simulink model "COSTEP_Auto"  (R2024b)
settings: Solver=FixedStepAuto  StartTime=0.0  StopTime=25  FixedStep=1/3600  RelTol=1e-3
model workspace (MAT data in the model file):
  AD : Simulink.Parameter (value not decoded)
  AG : Simulink.Parameter (value not decoded)
  AH : Simulink.Parameter (value not decoded)
  AV : Simulink.Parameter (value not decoded)
  AVP : Simulink.Parameter (value not decoded)
  BCHL : Simulink.Parameter (value not decoded)
  BCHV : Simulink.Parameter (value not decoded)
  BD : Simulink.Parameter (value not decoded)
  BG : Simulink.Parameter (value not decoded)
  BH : Simulink.Parameter (value not decoded)
  BVP : Simulink.Parameter (value not decoded)
  CD : Simulink.Parameter (value not decoded)
  CG : Simulink.Parameter (value not decoded)
  CH : Simulink.Parameter (value not decoded)
  CVP : Simulink.Parameter (value not decoded)
  ISV : Simulink.Parameter (value not decoded)
  XMW : Simulink.Parameter (value not decoded)
  XNS : Simulink.Parameter (value not decoded)
  XNS2 : Simulink.Parameter (value not decoded)
  XNS3 : Simulink.Parameter (value not decoded)
  XNSE : Simulink.Parameter (value not decoded)
values from neighbouring files (symbols this model uses):
  DD = SimData{4,1}{1,2}    [Auto_run_COSTEP.m]    (also in Run_COSTEP.m)
  G = SimData{2,1}(j,2)    [Auto_run_COSTEP.m]    (also in G.mat = [4243534565 7854912354 3456432354 1731738903 4346024432 5784; Run_COSTEP.m)
  IDV = SimData{3,1}(1:20,j)    [Auto_run_COSTEP.m]    (also in IDV.mat = [0 0 0 0 0 0 0 0 0 0 0 0 ... (812 elements, 28x29)]; Run_COSTEP.m = SimData{3,1}(1:28,j))
symbols that are objects in the model workspace (value not decoded): AD, AG, AH, AV, AVP, BD, BG, BH, BVP, CD, CG, CH, CVP, XMW, XNS, XNS2, XNS3, XNSE
undefined symbols (not defined in the file or in its folder): magnitude, msgbox, SETPT, XMEAS, XMV
libraries: mylib x304, dspindex x31
(part 12 of 13)

== system COSTEP_Auto/Random number generator/Stream Measurements SMEAS Gas analysis/If Action Subsystem3/Subsystem/Stream 13/Subsystem/TESUB6 XMNSEH ==
  G : Inport
  Process Noise I=1-12 G New : mylib/Process Noise I=1-12 G New  SystemSampleTime=-1  VariantActivationTime=update diagram  AllowFlexibleInterface=on  Latency=0  AutoFrameSizeCalculation=off
  XNSEH : Constant  Value=0.05
  XMNSEH : Outport  VectorParamsAs1DForOutWhenUnconnected=off
  G_NEW : Outport  Port=2  VectorParamsAs1DForOutWhenUnconnected=off
  wires:
  XNSEH/1 -> Process Noise I=1-12 G New/1
  Process Noise I=1-12 G New/1 -> XMNSEH/1
  G/1 -> Process Noise I=1-12 G New/2
  Process Noise I=1-12 G New/2 -> G_NEW/1

== system COSTEP_Auto/Random number generator/Stream Measurements SMEAS Gas analysis/If Action Subsystem3/Subsystem/Stream 2/Subsystem/TESUB6 XMNSEA ==
  G : Inport
  Process Noise I=1-12 G New : mylib/Process Noise I=1-12 G New  SystemSampleTime=-1  VariantActivationTime=update diagram  AllowFlexibleInterface=on  Latency=0  AutoFrameSizeCalculation=off
  XNSEA : Constant  Value=0.25
  XMNSEA : Outport  VectorParamsAs1DForOutWhenUnconnected=off
  G_NEW : Outport  Port=2  VectorParamsAs1DForOutWhenUnconnected=off
  wires:
  XNSEA/1 -> Process Noise I=1-12 G New/1
  Process Noise I=1-12 G New/1 -> XMNSEA/1
  G/1 -> Process Noise I=1-12 G New/2
  Process Noise I=1-12 G New/2 -> G_NEW/1

== system COSTEP_Auto/Random number generator/Stream Measurements SMEAS Gas analysis/If Action Subsystem3/Subsystem/Stream 2/Subsystem/TESUB6 XMNSEB ==
  G : Inport
  Process Noise I=1-12 G New : mylib/Process Noise I=1-12 G New  SystemSampleTime=-1  VariantActivationTime=update diagram  AllowFlexibleInterface=on  Latency=0  AutoFrameSizeCalculation=off
  XNSEB : Constant  Value=0.1
  XMNSEB : Outport  VectorParamsAs1DForOutWhenUnconnected=off
  G_NEW : Outport  Port=2  VectorParamsAs1DForOutWhenUnconnected=off
  wires:
  XNSEB/1 -> Process Noise I=1-12 G New/1
  Process Noise I=1-12 G New/1 -> XMNSEB/1
  G/1 -> Process Noise I=1-12 G New/2
  Process Noise I=1-12 G New/2 -> G_NEW/1

== system COSTEP_Auto/Random number generator/Stream Measurements SMEAS Gas analysis/If Action Subsystem3/Subsystem/Stream 2/Subsystem/TESUB6 XMNSEC ==
  G : Inport
  Process Noise I=1-12 G New : mylib/Process Noise I=1-12 G New  SystemSampleTime=-1  VariantActivationTime=update diagram  AllowFlexibleInterface=on  Latency=0  AutoFrameSizeCalculation=off
  XNSEC : Constant  Value=0.25
  XMNSEC : Outport  VectorParamsAs1DForOutWhenUnconnected=off
  G_NEW : Outport  Port=2  VectorParamsAs1DForOutWhenUnconnected=off
  wires:
  XNSEC/1 -> Process Noise I=1-12 G New/1
  Process Noise I=1-12 G New/1 -> XMNSEC/1
  G/1 -> Process Noise I=1-12 G New/2
  Process Noise I=1-12 G New/2 -> G_NEW/1

== system COSTEP_Auto/Random number generator/Stream Measurements SMEAS Gas analysis/If Action Subsystem3/Subsystem/Stream 2/Subsystem/TESUB6 XMNSED ==
  G : Inport
  Process Noise I=1-12 G New : mylib/Process Noise I=1-12 G New  SystemSampleTime=-1  VariantActivationTime=update diagram  AllowFlexibleInterface=on  Latency=0  AutoFrameSizeCalculation=off
  XNSED : Constant  Value=0.1
  XMNSED : Outport  VectorParamsAs1DForOutWhenUnconnected=off
  G_NEW : Outport  Port=2  VectorParamsAs1DForOutWhenUnconnected=off
  wires:
  XNSED/1 -> Process Noise I=1-12 G New/1
  Process Noise I=1-12 G New/1 -> XMNSED/1
  G/1 -> Process Noise I=1-12 G New/2
  Process Noise I=1-12 G New/2 -> G_NEW/1

== system COSTEP_Auto/Random number generator/Stream Measurements SMEAS Gas analysis/If Action Subsystem3/Subsystem/Stream 2/Subsystem/TESUB6 XMNSEE ==
  G : Inport
  Process Noise I=1-12 G New : mylib/Process Noise I=1-12 G New  SystemSampleTime=-1  VariantActivationTime=update diagram  AllowFlexibleInterface=on  Latency=0  AutoFrameSizeCalculation=off
  XNSEE : Constant  Value=0.25
  XMNSEE : Outport  VectorParamsAs1DForOutWhenUnconnected=off
  G_NEW : Outport  Port=2  VectorParamsAs1DForOutWhenUnconnected=off
  wires:
  XNSEE/1 -> Process Noise I=1-12 G New/1
  Process Noise I=1-12 G New/1 -> XMNSEE/1
  G/1 -> Process Noise I=1-12 G New/2
  Process Noise I=1-12 G New/2 -> G_NEW/1

== system COSTEP_Auto/Random number generator/Stream Measurements SMEAS Gas analysis/If Action Subsystem3/Subsystem/Stream 2/Subsystem/TESUB6 XMNSEF ==
  G : Inport
  Process Noise I=1-12 G New : mylib/Process Noise I=1-12 G New  SystemSampleTime=-1  VariantActivationTime=update diagram  AllowFlexibleInterface=on  Latency=0  AutoFrameSizeCalculation=off
  XNSEF : Constant  Value=0.025
  XMNSEF : Outport  VectorParamsAs1DForOutWhenUnconnected=off
  G_NEW : Outport  Port=2  VectorParamsAs1DForOutWhenUnconnected=off
  wires:
  XNSEF/1 -> Process Noise I=1-12 G New/1
  Process Noise I=1-12 G New/1 -> XMNSEF/1
  G/1 -> Process Noise I=1-12 G New/2
  Process Noise I=1-12 G New/2 -> G_NEW/1

== system COSTEP_Auto/Random number generator/Stream Measurements SMEAS Gas analysis/If Action Subsystem3/Subsystem/Stream 2/Subsystem/TESUB6 XMNSEG ==
  G : Inport
  Process Noise I=1-12 G New : mylib/Process Noise I=1-12 G New  SystemSampleTime=-1  VariantActivationTime=update diagram  AllowFlexibleInterface=on  Latency=0  AutoFrameSizeCalculation=off
  XNSEG : Constant  Value=0.05
  XMNSEG : Outport  VectorParamsAs1DForOutWhenUnconnected=off
  G_NEW : Outport  Port=2  VectorParamsAs1DForOutWhenUnconnected=off
  wires:
  XNSEG/1 -> Process Noise I=1-12 G New/1
  Process Noise I=1-12 G New/1 -> XMNSEG/1
  G/1 -> Process Noise I=1-12 G New/2
  Process Noise I=1-12 G New/2 -> G_NEW/1

== system COSTEP_Auto/Random number generator/Stream Measurements SMEAS Gas analysis/If Action Subsystem3/Subsystem/Stream 2/Subsystem/TESUB6 XMNSEH ==
  G : Inport
  Process Noise I=1-12 G New : mylib/Process Noise I=1-12 G New  SystemSampleTime=-1  VariantActivationTime=update diagram  AllowFlexibleInterface=on  Latency=0  AutoFrameSizeCalculation=off
  XNSEH : Constant  Value=0.05
  XMNSEH : Outport  VectorParamsAs1DForOutWhenUnconnected=off
  G_NEW : Outport  Port=2  VectorParamsAs1DForOutWhenUnconnected=off
  wires:
  XNSEH/1 -> Process Noise I=1-12 G New/1
  Process Noise I=1-12 G New/1 -> XMNSEH/1
  G/1 -> Process Noise I=1-12 G New/2
  Process Noise I=1-12 G New/2 -> G_NEW/1

== system COSTEP_Auto/Random number generator/Stream Measurements SMEAS Gas analysis/If Action Subsystem3/Subsystem/Stream 3/Subsystem/TESUB6 XMNSEA ==
  G : Inport
  Process Noise I=1-12 G New : mylib/Process Noise I=1-12 G New  SystemSampleTime=-1  VariantActivationTime=update diagram  AllowFlexibleInterface=on  Latency=0  AutoFrameSizeCalculation=off
  XNSEA : Constant  Value=0.25
  XMNSEA : Outport  VectorParamsAs1DForOutWhenUnconnected=off
  G_NEW : Outport  Port=2  VectorParamsAs1DForOutWhenUnconnected=off
  wires:
  XNSEA/1 -> Process Noise I=1-12 G New/1
  Process Noise I=1-12 G New/1 -> XMNSEA/1
  G/1 -> Process Noise I=1-12 G New/2
  Process Noise I=1-12 G New/2 -> G_NEW/1

== system COSTEP_Auto/Random number generator/Stream Measurements SMEAS Gas analysis/If Action Subsystem3/Subsystem/Stream 3/Subsystem/TESUB6 XMNSEB ==
  G : Inport
  Process Noise I=1-12 G New : mylib/Process Noise I=1-12 G New  SystemSampleTime=-1  VariantActivationTime=update diagram  AllowFlexibleInterface=on  Latency=0  AutoFrameSizeCalculation=off
  XNSEB : Constant  Value=0.1
  XMNSEB : Outport  VectorParamsAs1DForOutWhenUnconnected=off
  G_NEW : Outport  Port=2  VectorParamsAs1DForOutWhenUnconnected=off
  wires:
  XNSEB/1 -> Process Noise I=1-12 G New/1
  Process Noise I=1-12 G New/1 -> XMNSEB/1
  G/1 -> Process Noise I=1-12 G New/2
  Process Noise I=1-12 G New/2 -> G_NEW/1

== system COSTEP_Auto/Random number generator/Stream Measurements SMEAS Gas analysis/If Action Subsystem3/Subsystem/Stream 3/Subsystem/TESUB6 XMNSEC ==
  G : Inport
  Process Noise I=1-12 G New : mylib/Process Noise I=1-12 G New  SystemSampleTime=-1  VariantActivationTime=update diagram  AllowFlexibleInterface=on  Latency=0  AutoFrameSizeCalculation=off
  XNSEC : Constant  Value=0.25
  XMNSEC : Outport  VectorParamsAs1DForOutWhenUnconnected=off
  G_NEW : Outport  Port=2  VectorParamsAs1DForOutWhenUnconnected=off
  wires:
  XNSEC/1 -> Process Noise I=1-12 G New/1
  Process Noise I=1-12 G New/1 -> XMNSEC/1
  G/1 -> Process Noise I=1-12 G New/2
  Process Noise I=1-12 G New/2 -> G_NEW/1

== system COSTEP_Auto/Random number generator/Stream Measurements SMEAS Gas analysis/If Action Subsystem3/Subsystem/Stream 3/Subsystem/TESUB6 XMNSED ==
  G : Inport
  Process Noise I=1-12 G New : mylib/Process Noise I=1-12 G New  SystemSampleTime=-1  VariantActivationTime=update diagram  AllowFlexibleInterface=on  Latency=0  AutoFrameSizeCalculation=off
  XNSED : Constant  Value=0.1
  XMNSED : Outport  VectorParamsAs1DForOutWhenUnconnected=off
  G_NEW : Outport  Port=2  VectorParamsAs1DForOutWhenUnconnected=off
  wires:
  XNSED/1 -> Process Noise I=1-12 G New/1
  Process Noise I=1-12 G New/1 -> XMNSED/1
  G/1 -> Process Noise I=1-12 G New/2
  Process Noise I=1-12 G New/2 -> G_NEW/1

== system COSTEP_Auto/Random number generator/Stream Measurements SMEAS Gas analysis/If Action Subsystem3/Subsystem/Stream 3/Subsystem/TESUB6 XMNSEE ==
  G : Inport
  Process Noise I=1-12 G New : mylib/Process Noise I=1-12 G New  SystemSampleTime=-1  VariantActivationTime=update diagram  AllowFlexibleInterface=on  Latency=0  AutoFrameSizeCalculation=off
  XNSEE : Constant  Value=0.25
  XMNSEE : Outport  VectorParamsAs1DForOutWhenUnconnected=off
  G_NEW : Outport  Port=2  VectorParamsAs1DForOutWhenUnconnected=off
  wires:
  XNSEE/1 -> Process Noise I=1-12 G New/1
  Process Noise I=1-12 G New/1 -> XMNSEE/1
  G/1 -> Process Noise I=1-12 G New/2
  Process Noise I=1-12 G New/2 -> G_NEW/1

== system COSTEP_Auto/Random number generator/Stream Measurements SMEAS Gas analysis/If Action Subsystem3/Subsystem/Stream 3/Subsystem/TESUB6 XMNSEF ==
  G : Inport
  Process Noise I=1-12 G New : mylib/Process Noise I=1-12 G New  SystemSampleTime=-1  VariantActivationTime=update diagram  AllowFlexibleInterface=on  Latency=0  AutoFrameSizeCalculation=off
  XNSEF : Constant  Value=0.025
  XMNSEF : Outport  VectorParamsAs1DForOutWhenUnconnected=off
  G_NEW : Outport  Port=2  VectorParamsAs1DForOutWhenUnconnected=off
  wires:
  XNSEF/1 -> Process Noise I=1-12 G New/1
  Process Noise I=1-12 G New/1 -> XMNSEF/1
  G/1 -> Process Noise I=1-12 G New/2
  Process Noise I=1-12 G New/2 -> G_NEW/1

== system COSTEP_Auto/Random number generator/Stream Measurements SMEAS Gas analysis/If Action Subsystem3/Subsystem/Stream 3/Subsystem/TESUB6 XMNSEG ==
  G : Inport
  Process Noise I=1-12 G New : mylib/Process Noise I=1-12 G New  SystemSampleTime=-1  VariantActivationTime=update diagram  AllowFlexibleInterface=on  Latency=0  AutoFrameSizeCalculation=off
  XNSEG : Constant  Value=0.05
  XMNSEG : Outport  VectorParamsAs1DForOutWhenUnconnected=off
  G_NEW : Outport  Port=2  VectorParamsAs1DForOutWhenUnconnected=off
  wires:
  XNSEG/1 -> Process Noise I=1-12 G New/1
  Process Noise I=1-12 G New/1 -> XMNSEG/1
  G/1 -> Process Noise I=1-12 G New/2
  Process Noise I=1-12 G New/2 -> G_NEW/1

== system COSTEP_Auto/Random number generator/Stream Measurements SMEAS Gas analysis/If Action Subsystem3/Subsystem/Stream 3/Subsystem/TESUB6 XMNSEH ==
  G : Inport
  Process Noise I=1-12 G New : mylib/Process Noise I=1-12 G New  SystemSampleTime=-1  VariantActivationTime=update diagram  AllowFlexibleInterface=on  Latency=0  AutoFrameSizeCalculation=off
  XNSEH : Constant  Value=0.05
  XMNSEH : Outport  VectorParamsAs1DForOutWhenUnconnected=off
  G_NEW : Outport  Port=2  VectorParamsAs1DForOutWhenUnconnected=off
  wires:
  XNSEH/1 -> Process Noise I=1-12 G New/1
  Process Noise I=1-12 G New/1 -> XMNSEH/1
  G/1 -> Process Noise I=1-12 G New/2
  Process Noise I=1-12 G New/2 -> G_NEW/1

== system COSTEP_Auto/Random number generator/Stream Measurements SMEAS Gas analysis/If Action Subsystem3/Subsystem/Stream 4/Subsystem/TESUB6 XMNSEA ==
  G : Inport
  Process Noise I=1-12 G New : mylib/Process Noise I=1-12 G New  SystemSampleTime=-1  VariantActivationTime=update diagram  AllowFlexibleInterface=on  Latency=0  AutoFrameSizeCalculation=off
  XNSEA : Constant  Value=0.25
  XMNSEA : Outport  VectorParamsAs1DForOutWhenUnconnected=off
  G_NEW : Outport  Port=2  VectorParamsAs1DForOutWhenUnconnected=off
  wires:
  XNSEA/1 -> Process Noise I=1-12 G New/1
  Process Noise I=1-12 G New/1 -> XMNSEA/1
  G/1 -> Process Noise I=1-12 G New/2
  Process Noise I=1-12 G New/2 -> G_NEW/1

== system COSTEP_Auto/Random number generator/Stream Measurements SMEAS Gas analysis/If Action Subsystem3/Subsystem/Stream 4/Subsystem/TESUB6 XMNSEB ==
  G : Inport
  Process Noise I=1-12 G New : mylib/Process Noise I=1-12 G New  SystemSampleTime=-1  VariantActivationTime=update diagram  AllowFlexibleInterface=on  Latency=0  AutoFrameSizeCalculation=off
  XNSEB : Constant  Value=0.1
  XMNSEB : Outport  VectorParamsAs1DForOutWhenUnconnected=off
  G_NEW : Outport  Port=2  VectorParamsAs1DForOutWhenUnconnected=off
  wires:
  XNSEB/1 -> Process Noise I=1-12 G New/1
  Process Noise I=1-12 G New/1 -> XMNSEB/1
  G/1 -> Process Noise I=1-12 G New/2
  Process Noise I=1-12 G New/2 -> G_NEW/1

== system COSTEP_Auto/Random number generator/Stream Measurements SMEAS Gas analysis/If Action Subsystem3/Subsystem/Stream 4/Subsystem/TESUB6 XMNSEC ==
  G : Inport
  Process Noise I=1-12 G New : mylib/Process Noise I=1-12 G New  SystemSampleTime=-1  VariantActivationTime=update diagram  AllowFlexibleInterface=on  Latency=0  AutoFrameSizeCalculation=off
  XNSEC : Constant  Value=0.25
  XMNSEC : Outport  VectorParamsAs1DForOutWhenUnconnected=off
  G_NEW : Outport  Port=2  VectorParamsAs1DForOutWhenUnconnected=off
  wires:
  XNSEC/1 -> Process Noise I=1-12 G New/1
  Process Noise I=1-12 G New/1 -> XMNSEC/1
  G/1 -> Process Noise I=1-12 G New/2
  Process Noise I=1-12 G New/2 -> G_NEW/1

== system COSTEP_Auto/Random number generator/Stream Measurements SMEAS Gas analysis/If Action Subsystem3/Subsystem/Stream 4/Subsystem/TESUB6 XMNSED ==
  G : Inport
  Process Noise I=1-12 G New : mylib/Process Noise I=1-12 G New  SystemSampleTime=-1  VariantActivationTime=update diagram  AllowFlexibleInterface=on  Latency=0  AutoFrameSizeCalculation=off
  XNSED : Constant  Value=0.1
  XMNSED : Outport  VectorParamsAs1DForOutWhenUnconnected=off
  G_NEW : Outport  Port=2  VectorParamsAs1DForOutWhenUnconnected=off
  wires:
  XNSED/1 -> Process Noise I=1-12 G New/1
  Process Noise I=1-12 G New/1 -> XMNSED/1
  G/1 -> Process Noise I=1-12 G New/2
  Process Noise I=1-12 G New/2 -> G_NEW/1

== system COSTEP_Auto/Random number generator/Stream Measurements SMEAS Gas analysis/If Action Subsystem3/Subsystem/Stream 4/Subsystem/TESUB6 XMNSEE ==
  G : Inport
  Process Noise I=1-12 G New : mylib/Process Noise I=1-12 G New  SystemSampleTime=-1  VariantActivationTime=update diagram  AllowFlexibleInterface=on  Latency=0  AutoFrameSizeCalculation=off
  XNSEE : Constant  Value=0.25
  XMNSEE : Outport  VectorParamsAs1DForOutWhenUnconnected=off
  G_NEW : Outport  Port=2  VectorParamsAs1DForOutWhenUnconnected=off
  wires:
  XNSEE/1 -> Process Noise I=1-12 G New/1
  Process Noise I=1-12 G New/1 -> XMNSEE/1
  G/1 -> Process Noise I=1-12 G New/2
  Process Noise I=1-12 G New/2 -> G_NEW/1

== system COSTEP_Auto/Random number generator/Stream Measurements SMEAS Gas analysis/If Action Subsystem3/Subsystem/Stream 4/Subsystem/TESUB6 XMNSEF ==
  G : Inport
  Process Noise I=1-12 G New : mylib/Process Noise I=1-12 G New  SystemSampleTime=-1  VariantActivationTime=update diagram  AllowFlexibleInterface=on  Latency=0  AutoFrameSizeCalculation=off
  XNSEF : Constant  Value=0.025
  XMNSEF : Outport  VectorParamsAs1DForOutWhenUnconnected=off
  G_NEW : Outport  Port=2  VectorParamsAs1DForOutWhenUnconnected=off
  wires:
  XNSEF/1 -> Process Noise I=1-12 G New/1
  Process Noise I=1-12 G New/1 -> XMNSEF/1
  G/1 -> Process Noise I=1-12 G New/2
  Process Noise I=1-12 G New/2 -> G_NEW/1

== system COSTEP_Auto/Random number generator/Stream Measurements SMEAS Gas analysis/If Action Subsystem3/Subsystem/Stream 4/Subsystem/TESUB6 XMNSEG ==
  G : Inport
  Process Noise I=1-12 G New : mylib/Process Noise I=1-12 G New  SystemSampleTime=-1  VariantActivationTime=update diagram  AllowFlexibleInterface=on  Latency=0  AutoFrameSizeCalculation=off
  XNSEG : Constant  Value=0.05
  XMNSEG : Outport  VectorParamsAs1DForOutWhenUnconnected=off
  G_NEW : Outport  Port=2  VectorParamsAs1DForOutWhenUnconnected=off
  wires:
  XNSEG/1 -> Process Noise I=1-12 G New/1
  Process Noise I=1-12 G New/1 -> XMNSEG/1
  G/1 -> Process Noise I=1-12 G New/2
  Process Noise I=1-12 G New/2 -> G_NEW/1

== system COSTEP_Auto/Random number generator/Stream Measurements SMEAS Gas analysis/If Action Subsystem3/Subsystem/Stream 4/Subsystem/TESUB6 XMNSEH ==
  G : Inport
  Process Noise I=1-12 G New : mylib/Process Noise I=1-12 G New  SystemSampleTime=-1  VariantActivationTime=update diagram  AllowFlexibleInterface=on  Latency=0  AutoFrameSizeCalculation=off
  XNSEH : Constant  Value=0.05
  XMNSEH : Outport  VectorParamsAs1DForOutWhenUnconnected=off
  G_NEW : Outport  Port=2  VectorParamsAs1DForOutWhenUnconnected=off
  wires:
  XNSEH/1 -> Process Noise I=1-12 G New/1
  Process Noise I=1-12 G New/1 -> XMNSEH/1
  G/1 -> Process Noise I=1-12 G New/2
  Process Noise I=1-12 G New/2 -> G_NEW/1

== system COSTEP_Auto/Random number generator/Stream Measurements SMEAS Gas analysis/If Action Subsystem3/Subsystem/Stream 5/Subsystem/TESUB6 XMNSEA ==
  G : Inport
  Process Noise I=1-12 G New : mylib/Process Noise I=1-12 G New  SystemSampleTime=-1  VariantActivationTime=update diagram  AllowFlexibleInterface=on  Latency=0  AutoFrameSizeCalculation=off
  XNSEA : Constant  Value=0.25
  XMNSEA : Outport  VectorParamsAs1DForOutWhenUnconnected=off
  G_NEW : Outport  Port=2  VectorParamsAs1DForOutWhenUnconnected=off
  wires:
  XNSEA/1 -> Process Noise I=1-12 G New/1
  Process Noise I=1-12 G New/1 -> XMNSEA/1
  G/1 -> Process Noise I=1-12 G New/2
  Process Noise I=1-12 G New/2 -> G_NEW/1

== system COSTEP_Auto/Random number generator/Stream Measurements SMEAS Gas analysis/If Action Subsystem3/Subsystem/Stream 5/Subsystem/TESUB6 XMNSEB ==
  G : Inport
  Process Noise I=1-12 G New : mylib/Process Noise I=1-12 G New  SystemSampleTime=-1  VariantActivationTime=update diagram  AllowFlexibleInterface=on  Latency=0  AutoFrameSizeCalculation=off
  XNSEB : Constant  Value=0.1
  XMNSEB : Outport  VectorParamsAs1DForOutWhenUnconnected=off
  G_NEW : Outport  Port=2  VectorParamsAs1DForOutWhenUnconnected=off
  wires:
  XNSEB/1 -> Process Noise I=1-12 G New/1
  Process Noise I=1-12 G New/1 -> XMNSEB/1
  G/1 -> Process Noise I=1-12 G New/2
  Process Noise I=1-12 G New/2 -> G_NEW/1

== system COSTEP_Auto/Random number generator/Stream Measurements SMEAS Gas analysis/If Action Subsystem3/Subsystem/Stream 5/Subsystem/TESUB6 XMNSEC ==
  G : Inport
  Process Noise I=1-12 G New : mylib/Process Noise I=1-12 G New  SystemSampleTime=-1  VariantActivationTime=update diagram  AllowFlexibleInterface=on  Latency=0  AutoFrameSizeCalculation=off
  XNSEC : Constant  Value=0.25
  XMNSEC : Outport  VectorParamsAs1DForOutWhenUnconnected=off
  G_NEW : Outport  Port=2  VectorParamsAs1DForOutWhenUnconnected=off
  wires:
  XNSEC/1 -> Process Noise I=1-12 G New/1
  Process Noise I=1-12 G New/1 -> XMNSEC/1
  G/1 -> Process Noise I=1-12 G New/2
  Process Noise I=1-12 G New/2 -> G_NEW/1

== system COSTEP_Auto/Random number generator/Stream Measurements SMEAS Gas analysis/If Action Subsystem3/Subsystem/Stream 5/Subsystem/TESUB6 XMNSED ==
  G : Inport
  Process Noise I=1-12 G New : mylib/Process Noise I=1-12 G New  SystemSampleTime=-1  VariantActivationTime=update diagram  AllowFlexibleInterface=on  Latency=0  AutoFrameSizeCalculation=off
  XNSED : Constant  Value=0.1
  XMNSED : Outport  VectorParamsAs1DForOutWhenUnconnected=off
  G_NEW : Outport  Port=2  VectorParamsAs1DForOutWhenUnconnected=off
  wires:
  XNSED/1 -> Process Noise I=1-12 G New/1
  Process Noise I=1-12 G New/1 -> XMNSED/1
  G/1 -> Process Noise I=1-12 G New/2
  Process Noise I=1-12 G New/2 -> G_NEW/1

== system COSTEP_Auto/Random number generator/Stream Measurements SMEAS Gas analysis/If Action Subsystem3/Subsystem/Stream 5/Subsystem/TESUB6 XMNSEE ==
  G : Inport
  Process Noise I=1-12 G New : mylib/Process Noise I=1-12 G New  SystemSampleTime=-1  VariantActivationTime=update diagram  AllowFlexibleInterface=on  Latency=0  AutoFrameSizeCalculation=off
  XNSEE : Constant  Value=0.25
  XMNSEE : Outport  VectorParamsAs1DForOutWhenUnconnected=off
  G_NEW : Outport  Port=2  VectorParamsAs1DForOutWhenUnconnected=off
  wires:
  XNSEE/1 -> Process Noise I=1-12 G New/1
  Process Noise I=1-12 G New/1 -> XMNSEE/1
  G/1 -> Process Noise I=1-12 G New/2
  Process Noise I=1-12 G New/2 -> G_NEW/1

== system COSTEP_Auto/Random number generator/Stream Measurements SMEAS Gas analysis/If Action Subsystem3/Subsystem/Stream 5/Subsystem/TESUB6 XMNSEF ==
  G : Inport
  Process Noise I=1-12 G New : mylib/Process Noise I=1-12 G New  SystemSampleTime=-1  VariantActivationTime=update diagram  AllowFlexibleInterface=on  Latency=0  AutoFrameSizeCalculation=off
  XNSEF : Constant  Value=0.025
  XMNSEF : Outport  VectorParamsAs1DForOutWhenUnconnected=off
  G_NEW : Outport  Port=2  VectorParamsAs1DForOutWhenUnconnected=off
  wires:
  XNSEF/1 -> Process Noise I=1-12 G New/1
  Process Noise I=1-12 G New/1 -> XMNSEF/1
  G/1 -> Process Noise I=1-12 G New/2
  Process Noise I=1-12 G New/2 -> G_NEW/1

== system COSTEP_Auto/Random number generator/Stream Measurements SMEAS Gas analysis/If Action Subsystem3/Subsystem/Stream 5/Subsystem/TESUB6 XMNSEG ==
  G : Inport
  Process Noise I=1-12 G New : mylib/Process Noise I=1-12 G New  SystemSampleTime=-1  VariantActivationTime=update diagram  AllowFlexibleInterface=on  Latency=0  AutoFrameSizeCalculation=off
  XNSEG : Constant  Value=0.05
  XMNSEG : Outport  VectorParamsAs1DForOutWhenUnconnected=off
  G_NEW : Outport  Port=2  VectorParamsAs1DForOutWhenUnconnected=off
  wires:
  XNSEG/1 -> Process Noise I=1-12 G New/1
  Process Noise I=1-12 G New/1 -> XMNSEG/1
  G/1 -> Process Noise I=1-12 G New/2
  Process Noise I=1-12 G New/2 -> G_NEW/1

== system COSTEP_Auto/Random number generator/Stream Measurements SMEAS Gas analysis/If Action Subsystem3/Subsystem/Stream 5/Subsystem/TESUB6 XMNSEH ==
  G : Inport
  Process Noise I=1-12 G New : mylib/Process Noise I=1-12 G New  SystemSampleTime=-1  VariantActivationTime=update diagram  AllowFlexibleInterface=on  Latency=0  AutoFrameSizeCalculation=off
  XNSEH : Constant  Value=0.05
  XMNSEH : Outport  VectorParamsAs1DForOutWhenUnconnected=off
  G_NEW : Outport  Port=2  VectorParamsAs1DForOutWhenUnconnected=off
  wires:
  XNSEH/1 -> Process Noise I=1-12 G New/1
  Process Noise I=1-12 G New/1 -> XMNSEH/1
  G/1 -> Process Noise I=1-12 G New/2
  Process Noise I=1-12 G New/2 -> G_NEW/1

== system COSTEP_Auto/Random number generator/Stream Measurements SMEAS Gas analysis/If Action Subsystem3/Subsystem/Stream 6/Subsystem/TESUB6 XMNSEA ==
  G : Inport
  Process Noise I=1-12 G New : mylib/Process Noise I=1-12 G New  SystemSampleTime=-1  VariantActivationTime=update diagram  AllowFlexibleInterface=on  Latency=0  AutoFrameSizeCalculation=off
  XNSEA : Constant  Value=0.25
  XMNSEA : Outport  VectorParamsAs1DForOutWhenUnconnected=off
  G_NEW : Outport  Port=2  VectorParamsAs1DForOutWhenUnconnected=off
  wires:
  XNSEA/1 -> Process Noise I=1-12 G New/1
  Process Noise I=1-12 G New/1 -> XMNSEA/1
  G/1 -> Process Noise I=1-12 G New/2
  Process Noise I=1-12 G New/2 -> G_NEW/1

== system COSTEP_Auto/Random number generator/Stream Measurements SMEAS Gas analysis/If Action Subsystem3/Subsystem/Stream 6/Subsystem/TESUB6 XMNSEB ==
  G : Inport
  Process Noise I=1-12 G New : mylib/Process Noise I=1-12 G New  SystemSampleTime=-1  VariantActivationTime=update diagram  AllowFlexibleInterface=on  Latency=0  AutoFrameSizeCalculation=off
  XNSEB : Constant  Value=0.1
  XMNSEB : Outport  VectorParamsAs1DForOutWhenUnconnected=off
  G_NEW : Outport  Port=2  VectorParamsAs1DForOutWhenUnconnected=off
  wires:
  XNSEB/1 -> Process Noise I=1-12 G New/1
  Process Noise I=1-12 G New/1 -> XMNSEB/1
  G/1 -> Process Noise I=1-12 G New/2
  Process Noise I=1-12 G New/2 -> G_NEW/1

== system COSTEP_Auto/Random number generator/Stream Measurements SMEAS Gas analysis/If Action Subsystem3/Subsystem/Stream 6/Subsystem/TESUB6 XMNSEC ==
  G : Inport
  Process Noise I=1-12 G New : mylib/Process Noise I=1-12 G New  SystemSampleTime=-1  VariantActivationTime=update diagram  AllowFlexibleInterface=on  Latency=0  AutoFrameSizeCalculation=off
  XNSEC : Constant  Value=0.25
  XMNSEC : Outport  VectorParamsAs1DForOutWhenUnconnected=off
  G_NEW : Outport  Port=2  VectorParamsAs1DForOutWhenUnconnected=off
  wires:
  XNSEC/1 -> Process Noise I=1-12 G New/1
  Process Noise I=1-12 G New/1 -> XMNSEC/1
  G/1 -> Process Noise I=1-12 G New/2
  Process Noise I=1-12 G New/2 -> G_NEW/1

== system COSTEP_Auto/Random number generator/Stream Measurements SMEAS Gas analysis/If Action Subsystem3/Subsystem/Stream 6/Subsystem/TESUB6 XMNSED ==
  G : Inport
  Process Noise I=1-12 G New : mylib/Process Noise I=1-12 G New  SystemSampleTime=-1  VariantActivationTime=update diagram  AllowFlexibleInterface=on  Latency=0  AutoFrameSizeCalculation=off
  XNSED : Constant  Value=0.1
  XMNSED : Outport  VectorParamsAs1DForOutWhenUnconnected=off
  G_NEW : Outport  Port=2  VectorParamsAs1DForOutWhenUnconnected=off
  wires:
  XNSED/1 -> Process Noise I=1-12 G New/1
  Process Noise I=1-12 G New/1 -> XMNSED/1
  G/1 -> Process Noise I=1-12 G New/2
  Process Noise I=1-12 G New/2 -> G_NEW/1

== system COSTEP_Auto/Random number generator/Stream Measurements SMEAS Gas analysis/If Action Subsystem3/Subsystem/Stream 6/Subsystem/TESUB6 XMNSEE ==
  G : Inport
  Process Noise I=1-12 G New : mylib/Process Noise I=1-12 G New  SystemSampleTime=-1  VariantActivationTime=update diagram  AllowFlexibleInterface=on  Latency=0  AutoFrameSizeCalculation=off
  XNSEE : Constant  Value=0.25
  XMNSEE : Outport  VectorParamsAs1DForOutWhenUnconnected=off
  G_NEW : Outport  Port=2  VectorParamsAs1DForOutWhenUnconnected=off
  wires:
  XNSEE/1 -> Process Noise I=1-12 G New/1
  Process Noise I=1-12 G New/1 -> XMNSEE/1
  G/1 -> Process Noise I=1-12 G New/2
  Process Noise I=1-12 G New/2 -> G_NEW/1

== system COSTEP_Auto/Random number generator/Stream Measurements SMEAS Gas analysis/If Action Subsystem3/Subsystem/Stream 6/Subsystem/TESUB6 XMNSEF ==
  G : Inport
  Process Noise I=1-12 G New : mylib/Process Noise I=1-12 G New  SystemSampleTime=-1  VariantActivationTime=update diagram  AllowFlexibleInterface=on  Latency=0  AutoFrameSizeCalculation=off
  XNSEF : Constant  Value=0.025
  XMNSEF : Outport  VectorParamsAs1DForOutWhenUnconnected=off
  G_NEW : Outport  Port=2  VectorParamsAs1DForOutWhenUnconnected=off
  wires:
  XNSEF/1 -> Process Noise I=1-12 G New/1
  Process Noise I=1-12 G New/1 -> XMNSEF/1
  G/1 -> Process Noise I=1-12 G New/2
  Process Noise I=1-12 G New/2 -> G_NEW/1

== system COSTEP_Auto/Random number generator/Stream Measurements SMEAS Gas analysis/If Action Subsystem3/Subsystem/Stream 6/Subsystem/TESUB6 XMNSEG ==
  G : Inport
  Process Noise I=1-12 G New : mylib/Process Noise I=1-12 G New  SystemSampleTime=-1  VariantActivationTime=update diagram  AllowFlexibleInterface=on  Latency=0  AutoFrameSizeCalculation=off
  XNSEG : Constant  Value=0.05
  XMNSEG : Outport  VectorParamsAs1DForOutWhenUnconnected=off
  G_NEW : Outport  Port=2  VectorParamsAs1DForOutWhenUnconnected=off
  wires:
  XNSEG/1 -> Process Noise I=1-12 G New/1
  Process Noise I=1-12 G New/1 -> XMNSEG/1
  G/1 -> Process Noise I=1-12 G New/2
  Process Noise I=1-12 G New/2 -> G_NEW/1

== system COSTEP_Auto/Random number generator/Stream Measurements SMEAS Gas analysis/If Action Subsystem3/Subsystem/Stream 6/Subsystem/TESUB6 XMNSEH ==
  G : Inport
  Process Noise I=1-12 G New : mylib/Process Noise I=1-12 G New  SystemSampleTime=-1  VariantActivationTime=update diagram  AllowFlexibleInterface=on  Latency=0  AutoFrameSizeCalculation=off
  XNSEH : Constant  Value=0.05
  XMNSEH : Outport  VectorParamsAs1DForOutWhenUnconnected=off
  G_NEW : Outport  Port=2  VectorParamsAs1DForOutWhenUnconnected=off
  wires:
  XNSEH/1 -> Process Noise I=1-12 G New/1
  Process Noise I=1-12 G New/1 -> XMNSEH/1
  G/1 -> Process Noise I=1-12 G New/2
  Process Noise I=1-12 G New/2 -> G_NEW/1

== system COSTEP_Auto/Random number generator/Stream Measurements SMEAS Gas analysis/If Action Subsystem3/Subsystem/Stream 8/Subsystem/TESUB6 XMNSEA ==
  G : Inport
  Process Noise I=1-12 G New : mylib/Process Noise I=1-12 G New  SystemSampleTime=-1  VariantActivationTime=update diagram  AllowFlexibleInterface=on  Latency=0  AutoFrameSizeCalculation=off
  XNSEA : Constant  Value=0.25
  XMNSEA : Outport  VectorParamsAs1DForOutWhenUnconnected=off
  G_NEW : Outport  Port=2  VectorParamsAs1DForOutWhenUnconnected=off
  wires:
  XNSEA/1 -> Process Noise I=1-12 G New/1
  Process Noise I=1-12 G New/1 -> XMNSEA/1
  G/1 -> Process Noise I=1-12 G New/2
  Process Noise I=1-12 G New/2 -> G_NEW/1

== system COSTEP_Auto/Random number generator/Stream Measurements SMEAS Gas analysis/If Action Subsystem3/Subsystem/Stream 8/Subsystem/TESUB6 XMNSEB ==
  G : Inport
  Process Noise I=1-12 G New : mylib/Process Noise I=1-12 G New  SystemSampleTime=-1  VariantActivationTime=update diagram  AllowFlexibleInterface=on  Latency=0  AutoFrameSizeCalculation=off
  XNSEB : Constant  Value=0.1
  XMNSEB : Outport  VectorParamsAs1DForOutWhenUnconnected=off
  G_NEW : Outport  Port=2  VectorParamsAs1DForOutWhenUnconnected=off
  wires:
  XNSEB/1 -> Process Noise I=1-12 G New/1
  Process Noise I=1-12 G New/1 -> XMNSEB/1
  G/1 -> Process Noise I=1-12 G New/2
  Process Noise I=1-12 G New/2 -> G_NEW/1

== system COSTEP_Auto/Random number generator/Stream Measurements SMEAS Gas analysis/If Action Subsystem3/Subsystem/Stream 8/Subsystem/TESUB6 XMNSEC ==
  G : Inport
  Process Noise I=1-12 G New : mylib/Process Noise I=1-12 G New  SystemSampleTime=-1  VariantActivationTime=update diagram  AllowFlexibleInterface=on  Latency=0  AutoFrameSizeCalculation=off
  XNSEC : Constant  Value=0.25
  XMNSEC : Outport  VectorParamsAs1DForOutWhenUnconnected=off
  G_NEW : Outport  Port=2  VectorParamsAs1DForOutWhenUnconnected=off
  wires:
  XNSEC/1 -> Process Noise I=1-12 G New/1
  Process Noise I=1-12 G New/1 -> XMNSEC/1
  G/1 -> Process Noise I=1-12 G New/2
  Process Noise I=1-12 G New/2 -> G_NEW/1

== system COSTEP_Auto/Random number generator/Stream Measurements SMEAS Gas analysis/If Action Subsystem3/Subsystem/Stream 8/Subsystem/TESUB6 XMNSED ==
  G : Inport
  Process Noise I=1-12 G New : mylib/Process Noise I=1-12 G New  SystemSampleTime=-1  VariantActivationTime=update diagram  AllowFlexibleInterface=on  Latency=0  AutoFrameSizeCalculation=off
  XNSED : Constant  Value=0.1
  XMNSED : Outport  VectorParamsAs1DForOutWhenUnconnected=off
  G_NEW : Outport  Port=2  VectorParamsAs1DForOutWhenUnconnected=off
  wires:
  XNSED/1 -> Process Noise I=1-12 G New/1
  Process Noise I=1-12 G New/1 -> XMNSED/1
  G/1 -> Process Noise I=1-12 G New/2
  Process Noise I=1-12 G New/2 -> G_NEW/1

== system COSTEP_Auto/Random number generator/Stream Measurements SMEAS Gas analysis/If Action Subsystem3/Subsystem/Stream 8/Subsystem/TESUB6 XMNSEE ==
  G : Inport
  Process Noise I=1-12 G New : mylib/Process Noise I=1-12 G New  SystemSampleTime=-1  VariantActivationTime=update diagram  AllowFlexibleInterface=on  Latency=0  AutoFrameSizeCalculation=off
  XNSEE : Constant  Value=0.25
  XMNSEE : Outport  VectorParamsAs1DForOutWhenUnconnected=off
  G_NEW : Outport  Port=2  VectorParamsAs1DForOutWhenUnconnected=off
  wires:
  XNSEE/1 -> Process Noise I=1-12 G New/1
  Process Noise I=1-12 G New/1 -> XMNSEE/1
  G/1 -> Process Noise I=1-12 G New/2
  Process Noise I=1-12 G New/2 -> G_NEW/1

== system COSTEP_Auto/Random number generator/Stream Measurements SMEAS Gas analysis/If Action Subsystem3/Subsystem/Stream 8/Subsystem/TESUB6 XMNSEF ==
  G : Inport
  Process Noise I=1-12 G New : mylib/Process Noise I=1-12 G New  SystemSampleTime=-1  VariantActivationTime=update diagram  AllowFlexibleInterface=on  Latency=0  AutoFrameSizeCalculation=off
  XNSEF : Constant  Value=0.025
  XMNSEF : Outport  VectorParamsAs1DForOutWhenUnconnected=off
  G_NEW : Outport  Port=2  VectorParamsAs1DForOutWhenUnconnected=off
  wires:
  XNSEF/1 -> Process Noise I=1-12 G New/1
  Process Noise I=1-12 G New/1 -> XMNSEF/1
  G/1 -> Process Noise I=1-12 G New/2
  Process Noise I=1-12 G New/2 -> G_NEW/1

== system COSTEP_Auto/Random number generator/Stream Measurements SMEAS Gas analysis/If Action Subsystem3/Subsystem/Stream 8/Subsystem/TESUB6 XMNSEG ==
  G : Inport
  Process Noise I=1-12 G New : mylib/Process Noise I=1-12 G New  SystemSampleTime=-1  VariantActivationTime=update diagram  AllowFlexibleInterface=on  Latency=0  AutoFrameSizeCalculation=off
  XNSEG : Constant  Value=0.05
  XMNSEG : Outport  VectorParamsAs1DForOutWhenUnconnected=off
  G_NEW : Outport  Port=2  VectorParamsAs1DForOutWhenUnconnected=off
  wires:
  XNSEG/1 -> Process Noise I=1-12 G New/1
  Process Noise I=1-12 G New/1 -> XMNSEG/1
  G/1 -> Process Noise I=1-12 G New/2
  Process Noise I=1-12 G New/2 -> G_NEW/1

== system COSTEP_Auto/Random number generator/Stream Measurements SMEAS Gas analysis/If Action Subsystem3/Subsystem/Stream 8/Subsystem/TESUB6 XMNSEH ==
  G : Inport
  Process Noise I=1-12 G New : mylib/Process Noise I=1-12 G New  SystemSampleTime=-1  VariantActivationTime=update diagram  AllowFlexibleInterface=on  Latency=0  AutoFrameSizeCalculation=off
  XNSEH : Constant  Value=0.05
  XMNSEH : Outport  VectorParamsAs1DForOutWhenUnconnected=off
  G_NEW : Outport  Port=2  VectorParamsAs1DForOutWhenUnconnected=off
  wires:
  XNSEH/1 -> Process Noise I=1-12 G New/1
  Process Noise I=1-12 G New/1 -> XMNSEH/1
  G/1 -> Process Noise I=1-12 G New/2
  Process Noise I=1-12 G New/2 -> G_NEW/1

== system COSTEP_Auto/Random number generator/Stream Measurements SMEAS Gas analysis/If Action Subsystem3/Subsystem/Stream 9/Subsystem/TESUB6 XMNSEA ==
  G : Inport
  Process Noise I=1-12 G New : mylib/Process Noise I=1-12 G New  SystemSampleTime=-1  VariantActivationTime=update diagram  AllowFlexibleInterface=on  Latency=0  AutoFrameSizeCalculation=off
  XNSEA : Constant  Value=0.25
  XMNSEA : Outport  VectorParamsAs1DForOutWhenUnconnected=off
  G_NEW : Outport  Port=2  VectorParamsAs1DForOutWhenUnconnected=off
  wires:
  XNSEA/1 -> Process Noise I=1-12 G New/1
  Process Noise I=1-12 G New/1 -> XMNSEA/1
  G/1 -> Process Noise I=1-12 G New/2
  Process Noise I=1-12 G New/2 -> G_NEW/1

== system COSTEP_Auto/Random number generator/Stream Measurements SMEAS Gas analysis/If Action Subsystem3/Subsystem/Stream 9/Subsystem/TESUB6 XMNSEB ==
  G : Inport
  Process Noise I=1-12 G New : mylib/Process Noise I=1-12 G New  SystemSampleTime=-1  VariantActivationTime=update diagram  AllowFlexibleInterface=on  Latency=0  AutoFrameSizeCalculation=off
  XNSEB : Constant  Value=0.1
  XMNSEB : Outport  VectorParamsAs1DForOutWhenUnconnected=off
  G_NEW : Outport  Port=2  VectorParamsAs1DForOutWhenUnconnected=off
  wires:
  XNSEB/1 -> Process Noise I=1-12 G New/1
  Process Noise I=1-12 G New/1 -> XMNSEB/1
  G/1 -> Process Noise I=1-12 G New/2
  Process Noise I=1-12 G New/2 -> G_NEW/1

== system COSTEP_Auto/Random number generator/Stream Measurements SMEAS Gas analysis/If Action Subsystem3/Subsystem/Stream 9/Subsystem/TESUB6 XMNSEC ==
  G : Inport
  Process Noise I=1-12 G New : mylib/Process Noise I=1-12 G New  SystemSampleTime=-1  VariantActivationTime=update diagram  AllowFlexibleInterface=on  Latency=0  AutoFrameSizeCalculation=off
  XNSEC : Constant  Value=0.25
  XMNSEC : Outport  VectorParamsAs1DForOutWhenUnconnected=off
  G_NEW : Outport  Port=2  VectorParamsAs1DForOutWhenUnconnected=off
  wires:
  XNSEC/1 -> Process Noise I=1-12 G New/1
  Process Noise I=1-12 G New/1 -> XMNSEC/1
  G/1 -> Process Noise I=1-12 G New/2
  Process Noise I=1-12 G New/2 -> G_NEW/1

== system COSTEP_Auto/Random number generator/Stream Measurements SMEAS Gas analysis/If Action Subsystem3/Subsystem/Stream 9/Subsystem/TESUB6 XMNSED ==
  G : Inport
  Process Noise I=1-12 G New : mylib/Process Noise I=1-12 G New  SystemSampleTime=-1  VariantActivationTime=update diagram  AllowFlexibleInterface=on  Latency=0  AutoFrameSizeCalculation=off
  XNSED : Constant  Value=0.1
  XMNSED : Outport  VectorParamsAs1DForOutWhenUnconnected=off
  G_NEW : Outport  Port=2  VectorParamsAs1DForOutWhenUnconnected=off
  wires:
  XNSED/1 -> Process Noise I=1-12 G New/1
  Process Noise I=1-12 G New/1 -> XMNSED/1
  G/1 -> Process Noise I=1-12 G New/2
  Process Noise I=1-12 G New/2 -> G_NEW/1

== system COSTEP_Auto/Random number generator/Stream Measurements SMEAS Gas analysis/If Action Subsystem3/Subsystem/Stream 9/Subsystem/TESUB6 XMNSEE ==
  G : Inport
  Process Noise I=1-12 G New : mylib/Process Noise I=1-12 G New  SystemSampleTime=-1  VariantActivationTime=update diagram  AllowFlexibleInterface=on  Latency=0  AutoFrameSizeCalculation=off
  XNSEE : Constant  Value=0.25
  XMNSEE : Outport  VectorParamsAs1DForOutWhenUnconnected=off
  G_NEW : Outport  Port=2  VectorParamsAs1DForOutWhenUnconnected=off
  wires:
  XNSEE/1 -> Process Noise I=1-12 G New/1
  Process Noise I=1-12 G New/1 -> XMNSEE/1
  G/1 -> Process Noise I=1-12 G New/2
  Process Noise I=1-12 G New/2 -> G_NEW/1

== system COSTEP_Auto/Random number generator/Stream Measurements SMEAS Gas analysis/If Action Subsystem3/Subsystem/Stream 9/Subsystem/TESUB6 XMNSEF ==
  G : Inport
  Process Noise I=1-12 G New : mylib/Process Noise I=1-12 G New  SystemSampleTime=-1  VariantActivationTime=update diagram  AllowFlexibleInterface=on  Latency=0  AutoFrameSizeCalculation=off
  XNSEF : Constant  Value=0.025
  XMNSEF : Outport  VectorParamsAs1DForOutWhenUnconnected=off
  G_NEW : Outport  Port=2  VectorParamsAs1DForOutWhenUnconnected=off
  wires:
  XNSEF/1 -> Process Noise I=1-12 G New/1
  Process Noise I=1-12 G New/1 -> XMNSEF/1
  G/1 -> Process Noise I=1-12 G New/2
  Process Noise I=1-12 G New/2 -> G_NEW/1

== system COSTEP_Auto/Random number generator/Stream Measurements SMEAS Gas analysis/If Action Subsystem3/Subsystem/Stream 9/Subsystem/TESUB6 XMNSEG ==
  G : Inport
  Process Noise I=1-12 G New : mylib/Process Noise I=1-12 G New  SystemSampleTime=-1  VariantActivationTime=update diagram  AllowFlexibleInterface=on  Latency=0  AutoFrameSizeCalculation=off
  XNSEG : Constant  Value=0.05
  XMNSEG : Outport  VectorParamsAs1DForOutWhenUnconnected=off
  G_NEW : Outport  Port=2  VectorParamsAs1DForOutWhenUnconnected=off
  wires:
  XNSEG/1 -> Process Noise I=1-12 G New/1
  Process Noise I=1-12 G New/1 -> XMNSEG/1
  G/1 -> Process Noise I=1-12 G New/2
  Process Noise I=1-12 G New/2 -> G_NEW/1

== system COSTEP_Auto/Random number generator/Stream Measurements SMEAS Gas analysis/If Action Subsystem3/Subsystem/Stream 9/Subsystem/TESUB6 XMNSEH ==
  G : Inport
  Process Noise I=1-12 G New : mylib/Process Noise I=1-12 G New  SystemSampleTime=-1  VariantActivationTime=update diagram  AllowFlexibleInterface=on  Latency=0  AutoFrameSizeCalculation=off
  XNSEH : Constant  Value=0.05
  XMNSEH : Outport  VectorParamsAs1DForOutWhenUnconnected=off
  G_NEW : Outport  Port=2  VectorParamsAs1DForOutWhenUnconnected=off
  wires:
  XNSEH/1 -> Process Noise I=1-12 G New/1
  Process Noise I=1-12 G New/1 -> XMNSEH/1
  G/1 -> Process Noise I=1-12 G New/2
  Process Noise I=1-12 G New/2 -> G_NEW/1

== system COSTEP_Auto/Random number generator/Stream Measurements SMEAS Product analysis/If Action Subsystem3/Subsystem/Subsystem1/Subsystem/TESUB6 XMNSED ==
  G : Inport
  Process Noise I=1-12 G New : mylib/Process Noise I=1-12 G New  SystemSampleTime=-1  VariantActivationTime=update diagram  AllowFlexibleInterface=on  Latency=0  AutoFrameSizeCalculation=off
  XNS(37) : Constant  Value=0.01
  XMNS : Outport  VectorParamsAs1DForOutWhenUnconnected=off
  G_NEW : Outport  Port=2  VectorParamsAs1DForOutWhenUnconnected=off
  wires:
  XNS(37)/1 -> Process Noise I=1-12 G New/1
  Process Noise I=1-12 G New/1 -> XMNS/1
  G/1 -> Process Noise I=1-12 G New/2
  Process Noise I=1-12 G New/2 -> G_NEW/1

== system COSTEP_Auto/Random number generator/Stream Measurements SMEAS Product analysis/If Action Subsystem3/Subsystem/Subsystem1/Subsystem/TESUB6 XMNSEE ==
  G : Inport
  Process Noise I=1-12 G New : mylib/Process Noise I=1-12 G New  SystemSampleTime=-1  VariantActivationTime=update diagram  AllowFlexibleInterface=on  Latency=0  AutoFrameSizeCalculation=off
  XNS(38) : Constant  Value=0.01
  XMNS : Outport  VectorParamsAs1DForOutWhenUnconnected=off
  G_NEW : Outport  Port=2  VectorParamsAs1DForOutWhenUnconnected=off
  wires:
  XNS(38)/1 -> Process Noise I=1-12 G New/1
  Process Noise I=1-12 G New/1 -> XMNS/1
  G/1 -> Process Noise I=1-12 G New/2
  Process Noise I=1-12 G New/2 -> G_NEW/1

== system COSTEP_Auto/Random number generator/Stream Measurements SMEAS Product analysis/If Action Subsystem3/Subsystem/Subsystem1/Subsystem/TESUB6 XMNSEF ==
  G : Inport
  Process Noise I=1-12 G New : mylib/Process Noise I=1-12 G New  SystemSampleTime=-1  VariantActivationTime=update diagram  AllowFlexibleInterface=on  Latency=0  AutoFrameSizeCalculation=off
  XNS(39) : Constant  Value=0.01
  XMNS : Outport  VectorParamsAs1DForOutWhenUnconnected=off
  G_NEW : Outport  Port=2  VectorParamsAs1DForOutWhenUnconnected=off
  wires:
  XNS(39)/1 -> Process Noise I=1-12 G New/1
  Process Noise I=1-12 G New/1 -> XMNS/1
  G/1 -> Process Noise I=1-12 G New/2
  Process Noise I=1-12 G New/2 -> G_NEW/1

== system COSTEP_Auto/Random number generator/Stream Measurements SMEAS Product analysis/If Action Subsystem3/Subsystem/Subsystem1/Subsystem/TESUB6 XMNSEG ==
  G : Inport
  Process Noise I=1-12 G New : mylib/Process Noise I=1-12 G New  SystemSampleTime=-1  VariantActivationTime=update diagram  AllowFlexibleInterface=on  Latency=0  AutoFrameSizeCalculation=off
  XNS(40) : Constant  Value=0.5
  XMNS : Outport  VectorParamsAs1DForOutWhenUnconnected=off
  G_NEW : Outport  Port=2  VectorParamsAs1DForOutWhenUnconnected=off
  wires:
  XNS(40)/1 -> Process Noise I=1-12 G New/1
  Process Noise I=1-12 G New/1 -> XMNS/1
  G/1 -> Process Noise I=1-12 G New/2
  Process Noise I=1-12 G New/2 -> G_NEW/1

== system COSTEP_Auto/Random number generator/Stream Measurements SMEAS Product analysis/If Action Subsystem3/Subsystem/Subsystem1/Subsystem/TESUB6 XMNSEH ==
  G : Inport
  Process Noise I=1-12 G New : mylib/Process Noise I=1-12 G New  SystemSampleTime=-1  VariantActivationTime=update diagram  AllowFlexibleInterface=on  Latency=0  AutoFrameSizeCalculation=off
  XNS(41) : Constant  Value=0.5
  XMNS : Outport  VectorParamsAs1DForOutWhenUnconnected=off
  G_NEW : Outport  Port=2  VectorParamsAs1DForOutWhenUnconnected=off
  wires:
  XNS(41)/1 -> Process Noise I=1-12 G New/1
  Process Noise I=1-12 G New/1 -> XMNS/1
  G/1 -> Process Noise I=1-12 G New/2
  Process Noise I=1-12 G New/2 -> G_NEW/1

== system COSTEP_Auto/Random number generator/Stream Measurements SMEAS Product analysis/If Action Subsystem3/Subsystem/Subsystem2/Subsystem/TESUB6 XMNSED ==
  G : Inport
  Process Noise I=1-12 G New : mylib/Process Noise I=1-12 G New  SystemSampleTime=-1  VariantActivationTime=update diagram  AllowFlexibleInterface=on  Latency=0  AutoFrameSizeCalculation=off
  XNS(37) : Constant  Value=0.01
  XMNS : Outport  VectorParamsAs1DForOutWhenUnconnected=off
  G_NEW : Outport  Port=2  VectorParamsAs1DForOutWhenUnconnected=off
  wires:
  XNS(37)/1 -> Process Noise I=1-12 G New/1
  Process Noise I=1-12 G New/1 -> XMNS/1
  G/1 -> Process Noise I=1-12 G New/2
  Process Noise I=1-12 G New/2 -> G_NEW/1

== system COSTEP_Auto/Random number generator/Stream Measurements SMEAS Product analysis/If Action Subsystem3/Subsystem/Subsystem2/Subsystem/TESUB6 XMNSEE ==
  G : Inport
  Process Noise I=1-12 G New : mylib/Process Noise I=1-12 G New  SystemSampleTime=-1  VariantActivationTime=update diagram  AllowFlexibleInterface=on  Latency=0  AutoFrameSizeCalculation=off
  XNS(38) : Constant  Value=0.01
  XMNS : Outport  VectorParamsAs1DForOutWhenUnconnected=off
  G_NEW : Outport  Port=2  VectorParamsAs1DForOutWhenUnconnected=off
  wires:
  XNS(38)/1 -> Process Noise I=1-12 G New/1
  Process Noise I=1-12 G New/1 -> XMNS/1
  G/1 -> Process Noise I=1-12 G New/2
  Process Noise I=1-12 G New/2 -> G_NEW/1

== system COSTEP_Auto/Random number generator/Stream Measurements SMEAS Product analysis/If Action Subsystem3/Subsystem/Subsystem2/Subsystem/TESUB6 XMNSEF ==
  G : Inport
  Process Noise I=1-12 G New : mylib/Process Noise I=1-12 G New  SystemSampleTime=-1  VariantActivationTime=update diagram  AllowFlexibleInterface=on  Latency=0  AutoFrameSizeCalculation=off
  XNS(39) : Constant  Value=0.01
  XMNS : Outport  VectorParamsAs1DForOutWhenUnconnected=off
  G_NEW : Outport  Port=2  VectorParamsAs1DForOutWhenUnconnected=off
  wires:
  XNS(39)/1 -> Process Noise I=1-12 G New/1
  Process Noise I=1-12 G New/1 -> XMNS/1
  G/1 -> Process Noise I=1-12 G New/2
  Process Noise I=1-12 G New/2 -> G_NEW/1

== system COSTEP_Auto/Random number generator/Stream Measurements SMEAS Product analysis/If Action Subsystem3/Subsystem/Subsystem2/Subsystem/TESUB6 XMNSEG ==
  G : Inport
  Process Noise I=1-12 G New : mylib/Process Noise I=1-12 G New  SystemSampleTime=-1  VariantActivationTime=update diagram  AllowFlexibleInterface=on  Latency=0  AutoFrameSizeCalculation=off
  XNS(40) : Constant  Value=0.5
  XMNS : Outport  VectorParamsAs1DForOutWhenUnconnected=off
  G_NEW : Outport  Port=2  VectorParamsAs1DForOutWhenUnconnected=off
  wires:
  XNS(40)/1 -> Process Noise I=1-12 G New/1
  Process Noise I=1-12 G New/1 -> XMNS/1
  G/1 -> Process Noise I=1-12 G New/2
  Process Noise I=1-12 G New/2 -> G_NEW/1

== system COSTEP_Auto/Random number generator/Stream Measurements SMEAS Product analysis/If Action Subsystem3/Subsystem/Subsystem2/Subsystem/TESUB6 XMNSEH ==
  G : Inport
  Process Noise I=1-12 G New : mylib/Process Noise I=1-12 G New  SystemSampleTime=-1  VariantActivationTime=update diagram  AllowFlexibleInterface=on  Latency=0  AutoFrameSizeCalculation=off
  XNS(41) : Constant  Value=0.5
  XMNS : Outport  VectorParamsAs1DForOutWhenUnconnected=off
  G_NEW : Outport  Port=2  VectorParamsAs1DForOutWhenUnconnected=off
  wires:
  XNS(41)/1 -> Process Noise I=1-12 G New/1
  Process Noise I=1-12 G New/1 -> XMNS/1
  G/1 -> Process Noise I=1-12 G New/2
  Process Noise I=1-12 G New/2 -> G_NEW/1

== matlab function COSTEP_Auto/Random number generator/Stream Measurements SMEAS/MATLAB Function ==
  data: XNSE input; GE output; GE input; ISD input; Time input; XMNSE output
function [GE,XMNSE] = ProcessNoise(XNSE,GE,ISD,Time)

X =zeros(24,1);
RN=zeros(24*12+1,1);
RN(1,1)=GE;
TESUB7 = zeros(12,24);

if Time > 0.0 && ISD == 0

    for I=1:24
        
    TESUB7_value = zeros(1,24);
    
        for It =1:12
    
            RN((12*I-11+It),1) = mod(RN((12*I-11+It-1),1) * 9228907,4294967296);
                if It >= 0
                    TESUB7_value(I) = RN((12*I-11+It),1) / 4294967296;
                else
                    TESUB7_value(I) = 2 * RN((12*I-11+It),1) / 4294967296 - 1;
                end
            TESUB7(It,I)=TESUB7_value(I); 
            X(I) = X(I) + TESUB7(It,I);
        end 
    
        X(I) = (X(I) - 6) * XNSE(I,1);
        XMNSE = X;
    end 
    
    GE = RN(end);
    
else
    XMNSE = zeros(24,1);
    GE = RN(1,1);
end
